simulink model "SLIPquadold"  (R2015a)
settings: Solver=ode45  StartTime=0.0  StopTime=50  MaxStep=1e-3  RelTol=1e-4  AbsTol=1e-6
values from neighbouring files (symbols this model uses):
  a0 = 68*pi/180    (= 1.18682389136)    [SLIPquad_params.m]
  dt0 = deg2rad(0)    [SLIPquad_params.m]
  dx0 = 4.5    [SLIPquad_params.m]
  dy0 = 0    [SLIPquad_params.m]
  g = 9.81    [SLIPquad_params.m]
  J = 4.58    [SLIPquad_params.m]
  Jleg = mfoot*l0^2    (= 1.16)    [SLIPquad_params.m]
  k = 10000    [SLIPquad_params.m]
  L = 0.5    [SLIPquad_params.m]
  l0 = 1    [SLIPquad_params.m]
  m = 80    [SLIPquad_params.m]
  t0 = 0*pi/180    (= 0)    [SLIPquad_params.m]
  x0 = 0    [SLIPquad_params.m]
  xrb0 = -l0*cos(a0) + L*cos(t0)    [SLIPquad_params.m]
  xrf0 = -l0*cos(a0) - L*cos(t0)    [SLIPquad_params.m]
  y0 = 1    [SLIPquad_params.m]
  yrb0 = l0*sin(a0) + L*sin(t0)    [SLIPquad_params.m]
  yrf0 = l0*sin(a0) - L*sin(t0)    [SLIPquad_params.m]
libraries: simulink_extras x2
settings Model: Creator=hgeyer  LastModifiedBy=Joe
settings DataIOCC: LimitDataPoints=off  SignalLoggingSaveFormat=ModelDataLogs
settings OptimizationCC: ExpressionDepthLimit=2147483647
settings DebuggingCC: UnderspecifiedInitializationDetection=Classic  MergeDetectMultiDrivingBlocksExec=none  SolverPrmCheckMsg=warning  FcnCallInpInsideContextMsg=EnableAllAsWarning  StateNameClashWarn=warning

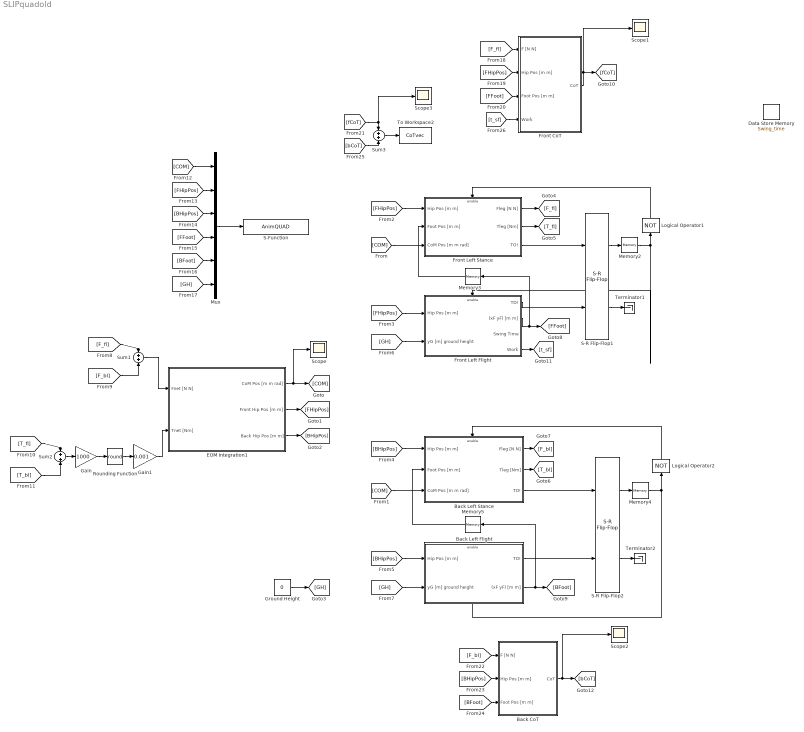
== system SLIPquadold ==
  Back CoT : Subsystem
  Back Left Flight : Subsystem
  Back Left Stance : Subsystem
  Data Store Memory : DataStoreMemory  DataStoreName=Swing_time  ReadBeforeWriteMsg=warning  WriteAfterWriteMsg=warning  WriteAfterReadMsg=warning
  EOM Integration1 : Subsystem
  Front CoT : Subsystem
  Front Left Flight : Subsystem
  Front Left Stance : Subsystem
  Gain : Gain  Gain=1000
  Gain1 : Gain  Gain=0.001
  Ground Height : Constant  Value=0
  Logical Operator1 : Logic  Operator=NOT  AllPortsSameDT=off  OutDataTypeStr=boolean
  Logical Operator2 : Logic  Operator=NOT  AllPortsSameDT=off  OutDataTypeStr=boolean
  Memory2 : Memory  X0=1
  Memory3 : Memory  X0=[(x0 - xrf0) (y0 - yrf0) ]
  Memory4 : Memory  X0=1
  Memory5 : Memory  X0=[(x0 - xrb0) (y0 - yrb0)]
  Mux : Mux  Inputs=6
  Rounding Function : Rounding  Operator=round
  S-Function : S-Function  FunctionName=AnimQUAD  Parameters=0.005
  S-R Flip-Flop1 : simulink_extras/Flip Flops/S-R Flip-Flop  initial_condition=1
  S-R Flip-Flop2 : simulink_extras/Flip Flops/S-R Flip-Flop  initial_condition=1
  Scope{,1..3} (4 alike) : Scope
      Scope2 settings: SaveName=ScopeData6
      Scope3 settings: SaveName=ScopeData7
  Sum1 : Sum  Inputs=+|+
  Sum2 : Sum  Inputs=+|+
  Sum3 : Sum  Inputs=+|+
  Terminator1 : Terminator
  Terminator2 : Terminator
  To Workspace2 : ToWorkspace  VariableName=CoTvec  SampleTime=-1
  wires:
  Front Left Stance/3(TO!) -> S-R Flip-Flop1/1
  S-R Flip-Flop1/1 -> Memory2/1
  Front Left Flight/1(TD!) -> S-R Flip-Flop1/2
  Memory2/1 -> Front Left Flight/Enable, Logical Operator1/1
  Logical Operator1/1 -> Front Left Stance/Enable
  S-R Flip-Flop1/2 -> Terminator1/1
  Front Left Flight/2((xF yF) [m m]) -> [FFoot], Memory3/1
  Memory3/1 -> Front Left Stance/2(Foot Pos [m m])
  Back Left Stance/3(TO!) -> S-R Flip-Flop2/1
  S-R Flip-Flop2/1 -> Memory4/1
  Back Left Flight/1(TO!) -> S-R Flip-Flop2/2
  Memory4/1 -> Back Left Flight/Enable, Logical Operator2/1
  Logical Operator2/1 -> Back Left Stance/Enable
  S-R Flip-Flop2/2 -> Terminator2/1
  [GH] -> Back Left Flight/2(yG [m] ground height)
  Back Left Flight/2((xF yF) [m m]) -> [BFoot], Memory5/1
  Memory5/1 -> Back Left Stance/2(Foot Pos [m m])
  Ground Height/1 -> [GH]
  [GH] -> Front Left Flight/2(yG [m] ground height)
  Front Left Stance/1(Fleg [N N]) -> [F_fl]
  Front Left Stance/2(Tleg [Nm]) -> [T_fl]
  Back Left Stance/1(Fleg [N N]) -> [F_bl]
  Back Left Stance/2(Tleg [Nm]) -> [T_bl]
  [F_fl] -> Sum1/1
  [F_bl] -> Sum1/2
  [T_fl] -> Sum2/1
  [T_bl] -> Sum2/2
  Sum1/1 -> EOM Integration1/1(Fnet [N N])
  EOM Integration1/1(CoM Pos [m m rad]) -> Scope/1, [COM]
  EOM Integration1/2(Front Hip Pos [m m]) -> [FHipPos]
  EOM Integration1/3(Back Hip Pos [m m]) -> [BHipPos]
  [FHipPos] -> Front Left Stance/1(Hip Pos [m m])
  [FHipPos] -> Front Left Flight/1(Hip Pos [m m])
  [BHipPos] -> Back Left Stance/1(Hip Pos [m m])
  [BHipPos] -> Back Left Flight/1(Hip Pos [m m])
  [COM] -> Front Left Stance/3(CoM Pos [m m rad])
  [COM] -> Back Left Stance/3(CoM Pos [m m rad])
  Sum2/1 -> Gain/1
  Gain1/1 -> EOM Integration1/2(Tnet [Nm])
  Gain/1 -> Rounding Function/1
  Rounding Function/1 -> Gain1/1
  Mux/1 -> S-Function/1
  [COM] -> Mux/1
  [FHipPos] -> Mux/2
  [BHipPos] -> Mux/3
  [FFoot] -> Mux/4
  [BFoot] -> Mux/5
  [GH] -> Mux/6
  [F_fl] -> Front CoT/1(F [N N])
  [FHipPos] -> Front CoT/2(Hip Pos [m m])
  [FFoot] -> Front CoT/3(Foot Pos [m m])
  Front CoT/1(CoT) -> [fCoT], Scope1/1
  [F_bl] -> Back CoT/1(F [N N])
  [BHipPos] -> Back CoT/2(Hip Pos [m m])
  [BFoot] -> Back CoT/3(Foot Pos [m m])
  Back CoT/1(CoT) -> [bCoT], Scope2/1
  [fCoT] -> Scope3/1, Sum3/1
  [bCoT] -> Sum3/2
  Sum3/1 -> To Workspace2/1
  [t_sf] -> Front CoT/4(Work)
  Front Left Flight/4(Work) -> [t_sf]

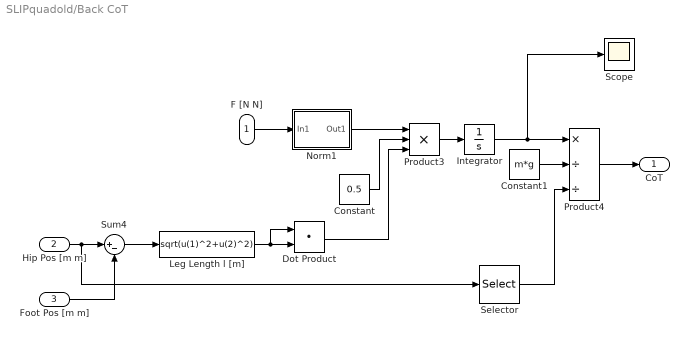
== system SLIPquadold/Back CoT ==
  F [N N] : Inport
  Hip Pos [m m] : Inport  Port=2
  Foot Pos [m m] : Inport  Port=3
  Constant : Constant  Value=0.5
  Constant1 : Constant  Value=m*g
  Dot Product : DotProduct  InputSameDT=on  OutDataTypeStr=Inherit: Inherit via internal rule
  Integrator : Integrator
  Leg Length l [m] : Fcn  Expr=sqrt(u(1)^2+u(2)^2)
  Norm1 : Subsystem
  Product3 : Product  Inputs=3
  Product4 : Product  Inputs=*//
  Scope : Scope
      settings: SaveName=ScopeData3
  Selector : Selector  InputPortWidth=2  Indices=[1]
  Sum4 : Sum  Inputs=|+-
  CoT : Outport
  wires:
  Constant/1 -> Product3/2
  Constant1/1 -> Product4/2
  Norm1/1(Out1) -> Product3/1
  Dot Product/1 -> Product3/3
  F [N N]/1 -> Norm1/1(In1)
  Leg Length l [m]/1 -> Dot Product/1, Dot Product/2
  Product4/1 -> CoT/1
  Product3/1 -> Integrator/1
  Selector/1 -> Product4/3
  Integrator/1 -> Scope/1, Product4/1
  Sum4/1 -> Leg Length l [m]/1
  Foot Pos [m m]/1 -> Sum4/2
  Hip Pos [m m]/1 -> Selector/1, Sum4/1

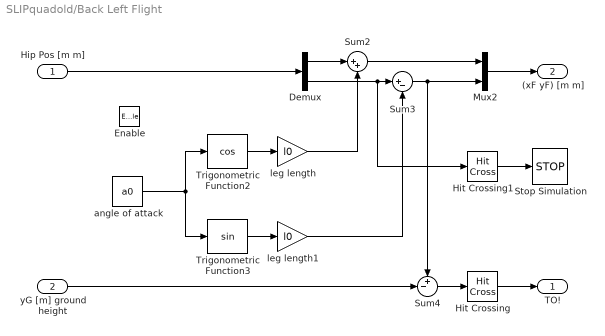
== system SLIPquadold/Back Left Flight ==
  Hip Pos [m m] : Inport
  yG [m] ground height : Inport  Port=2
  Enable : EnablePort  StatesWhenEnabling=reset
  Demux : Demux  Outputs=2
  Hit Crossing : HitCross  HitCrossingDirection=falling
  Hit Crossing1 : HitCross  HitCrossingDirection=falling
  Mux2 : Mux  Inputs=2
  Stop Simulation : Stop
  Sum2 : Sum  Inputs=|++
  Sum3 : Sum  Inputs=|+-
  Sum4 : Sum  Inputs=+-|
  Trigonometric Function2 : Trigonometry  Operator=cos
  Trigonometric Function3 : Trigonometry
  angle of attack : Constant  Value=a0
  leg length : Gain  Gain=l0
  leg length1 : Gain  Gain=l0
  TO! : Outport  OutputWhenDisabled=reset  InitialOutput=0
      settings: AttributesFormatString=%<OutputWhenDisabled>
  (xF yF) [m m] : Outport  Port=2  InitialOutput=[0 0]
      settings: AttributesFormatString=%<OutputWhenDisabled>
  wires:
  Hit Crossing/1 -> TO!/1
  Demux/2 -> Hit Crossing1/1, Sum3/1
  Demux/1 -> Sum2/1
  angle of attack/1 -> Trigonometric Function3/1, Trigonometric Function2/1
  Trigonometric Function2/1 -> leg length/1
  Trigonometric Function3/1 -> leg length1/1
  Hip Pos [m m]/1 -> Demux/1
  leg length/1 -> Sum2/2
  leg length1/1 -> Sum3/2
  Sum3/1 -> Mux2/2, Sum4/1
  Sum2/1 -> Mux2/1
  Mux2/1 -> (xF yF) [m m]/1
  yG [m] ground height/1 -> Sum4/2
  Sum4/1 -> Hit Crossing/1
  Hit Crossing1/1 -> Stop Simulation/1

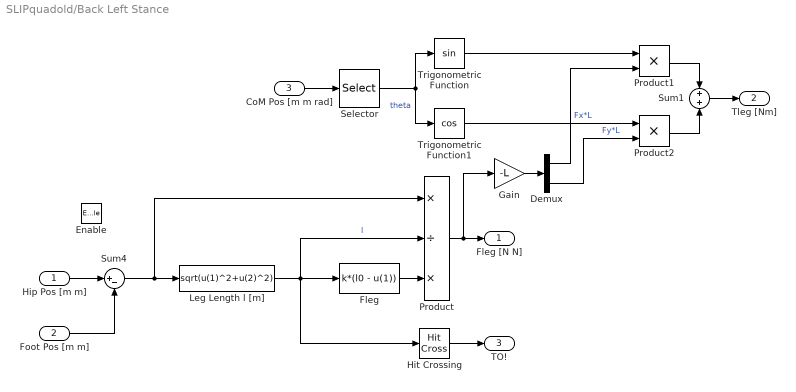
== system SLIPquadold/Back Left Stance ==
  Hip Pos [m m] : Inport
  Foot Pos [m m] : Inport  Port=2
  CoM Pos [m m rad] : Inport  Port=3
  Enable : EnablePort  StatesWhenEnabling=reset
  Demux : Demux  Outputs=2
  Fleg : Fcn  Expr=k*(l0 - u(1))
  Gain : Gain  Gain=-L
  Hit Crossing : HitCross  HitCrossingOffset=l0  HitCrossingDirection=rising
  Leg Length l [m] : Fcn  Expr=sqrt(u(1)^2+u(2)^2)
  Product : Product  Inputs=*/*
  Product1 : Product
  Product2 : Product
  Selector : Selector  InputPortWidth=3  Indices=[3]
  Sum1 : Sum  Inputs=+|+
  Sum4 : Sum  Inputs=|+-
  Trigonometric Function : Trigonometry
  Trigonometric Function1 : Trigonometry  Operator=cos
  Fleg [N N] : Outport  OutputWhenDisabled=reset  InitialOutput=[0 0]
      settings: AttributesFormatString=%<OutputWhenDisabled>
  Tleg [Nm] : Outport  Port=2  OutputWhenDisabled=reset  InitialOutput=[0]
      settings: AttributesFormatString=%<OutputWhenDisabled>
  TO! : Outport  Port=3  OutputWhenDisabled=reset  InitialOutput=[0]
      settings: AttributesFormatString=%<OutputWhenDisabled>
  wires:
  Sum1/1 -> Tleg [Nm]/1
  Product1/1 -> Sum1/1
  Product2/1 -> Sum1/2
  Gain/1 -> Demux/1
  Demux/2 -> Product2/2  "Fy*L"
  Demux/1 -> Product1/2  "Fx*L"
  Trigonometric Function/1 -> Product1/1
  Trigonometric Function1/1 -> Product2/1
  Selector/1 -> Trigonometric Function/1, Trigonometric Function1/1  "theta"
  CoM Pos [m m rad]/1 -> Selector/1
  Foot Pos [m m]/1 -> Sum4/2
  Hip Pos [m m]/1 -> Sum4/1
  Hit Crossing/1 -> TO!/1
  Product/1 -> Fleg [N N]/1, Gain/1
  Fleg/1 -> Product/3
  Leg Length l [m]/1 -> Hit Crossing/1, Product/2, Fleg/1  "l"
  Sum4/1 -> Leg Length l [m]/1, Product/1

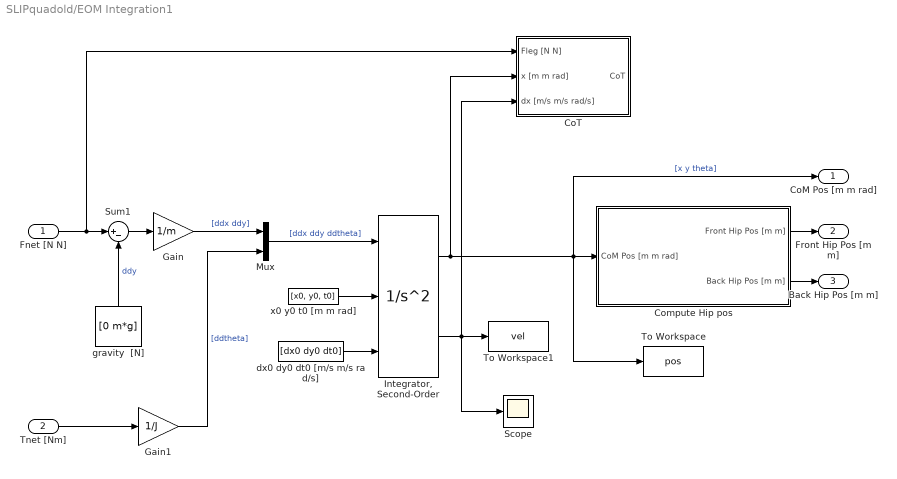
== system SLIPquadold/EOM Integration1 ==
  Fnet [N N] : Inport
  Tnet [Nm] : Inport  Port=2
  CoT : Subsystem
  Compute Hip pos : Subsystem
  Gain : Gain  Gain=1/m
  Gain1 : Gain  Gain=1/J
  "Integrator, Second-Order" : SecondOrderIntegrator  ICSourceX=external  ICSourceDXDT=external
  Mux : Mux  Inputs=2
  Scope : Scope
      settings: TimeRange=3.298211913921595  YMin=-10  YMax=10  SaveName=ScopeData2
  Sum1 : Sum  Inputs=|+-
  To Workspace : ToWorkspace  VariableName=pos  SampleTime=-1
  To Workspace1 : ToWorkspace  VariableName=vel  SampleTime=-1
  dx0 dy0 dt0 [m/s m/s ra d/s] : Constant  Value=[dx0 dy0 dt0]
  gravity  [N] : Constant  Value=[0 m*g]
  x0 y0 t0 [m m rad] : Constant  Value=[x0, y0, t0]
  CoM Pos [m m rad] : Outport
  Front Hip Pos [m m] : Outport  Port=2
  Back Hip Pos [m m] : Outport  Port=3
  wires:
  "Integrator, Second-Order"/2 -> CoT/3(dx [m/s m/s rad/s]), Scope/1, To Workspace1/1
  Compute Hip pos/1(Front Hip Pos [m m]) -> Front Hip Pos [m m]/1
  "Integrator, Second-Order"/1 -> CoT/2(x [m m rad]), CoM Pos [m m rad]/1, Compute Hip pos/1(CoM Pos [m m rad]), To Workspace/1  "[x y theta]"
  Tnet [Nm]/1 -> Gain1/1
  Gain1/1 -> Mux/2  "[ddtheta]"
  Mux/1 -> "Integrator, Second-Order"/1  "[ddx ddy ddtheta]"
  dx0 dy0 dt0 [m/s m/s ra d/s]/1 -> "Integrator, Second-Order"/3
  Fnet [N N]/1 -> CoT/1(Fleg [N N]), Sum1/1
  Gain/1 -> Mux/1  "[ddx ddy]"
  x0 y0 t0 [m m rad]/1 -> "Integrator, Second-Order"/2
  gravity  [N]/1 -> Sum1/2  "ddy"
  Sum1/1 -> Gain/1
  Compute Hip pos/2(Back Hip Pos [m m]) -> Back Hip Pos [m m]/1

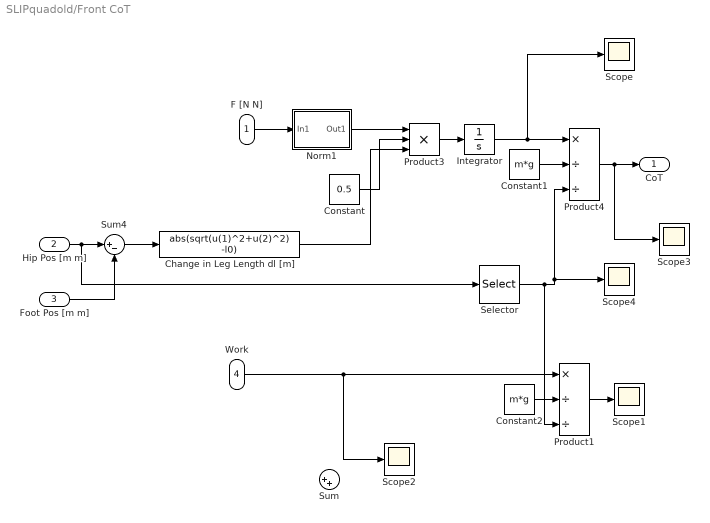
== system SLIPquadold/Front CoT ==
  F [N N] : Inport
  Hip Pos [m m] : Inport  Port=2
  Foot Pos [m m] : Inport  Port=3
  Work : Inport  Port=4
  Change in Leg Length dl [m] : Fcn  Expr=abs(sqrt(u(1)^2+u(2)^2) -l0)
  Constant : Constant  Value=0.5
  Constant1 : Constant  Value=m*g
  Constant2 : Constant  Value=m*g
  Integrator : Integrator
  Norm1 : Subsystem
  Product1 : Product  Inputs=*//
  Product3 : Product  Inputs=3
  Product4 : Product  Inputs=*//
  Scope{,1..4} (5 alike) : Scope
      Scope settings: YMin=2000  YMax=6000  SaveName=ScopeData3
      Scope1 settings: SaveName=ScopeData8
      Scope2 settings: SaveName=ScopeData9
      Scope3 settings: YMin=0.0443  YMax=0.04445  SaveName=ScopeData10
      Scope4 settings: YMin=2000  YMax=6000  SaveName=ScopeData12
  Selector : Selector  InputPortWidth=2  Indices=[1]
  Sum : Sum  Inputs=|++
  Sum4 : Sum  Inputs=|+-
  CoT : Outport
  wires:
  Constant/1 -> Product3/2
  Constant1/1 -> Product4/2
  Norm1/1(Out1) -> Product3/1
  F [N N]/1 -> Norm1/1(In1)
  Product4/1 -> Scope3/1, CoT/1
  Product3/1 -> Integrator/1
  Selector/1 -> Product1/3, Product4/3, Scope4/1
  Integrator/1 -> Scope/1, Product4/1
  Sum4/1 -> Change in Leg Length dl [m]/1
  Foot Pos [m m]/1 -> Sum4/2
  Hip Pos [m m]/1 -> Selector/1, Sum4/1
  Constant2/1 -> Product1/2
  Product1/1 -> Scope1/1
  Work/1 -> Product1/1, Scope2/1
  Change in Leg Length dl [m]/1 -> Product3/3

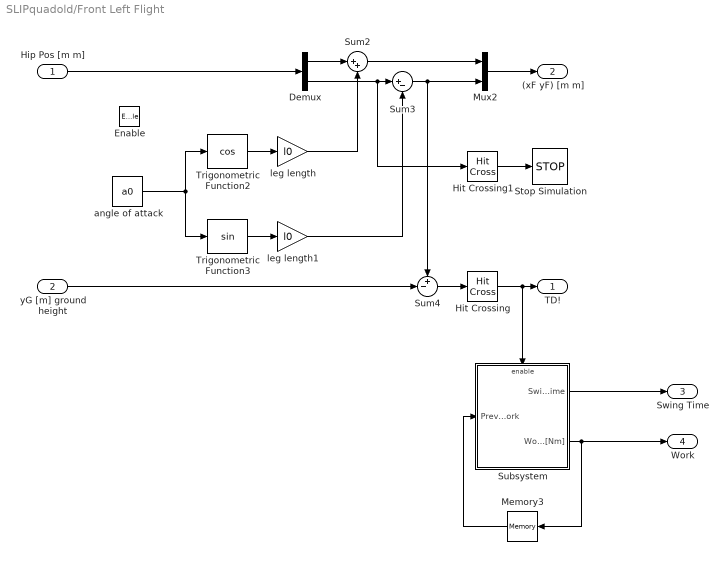
== system SLIPquadold/Front Left Flight ==
  Hip Pos [m m] : Inport
  yG [m] ground height : Inport  Port=2
  Enable : EnablePort  StatesWhenEnabling=reset
  Demux : Demux  Outputs=2
  Hit Crossing : HitCross  HitCrossingDirection=falling
  Hit Crossing1 : HitCross  HitCrossingDirection=falling
  Memory3 : Memory  X0=[(x0 - xrf0) (y0 - yrf0) ]
  Mux2 : Mux  Inputs=2
  Stop Simulation : Stop
  Subsystem : Subsystem
  Sum2 : Sum  Inputs=|++
  Sum3 : Sum  Inputs=|+-
  Sum4 : Sum  Inputs=+-|
  Trigonometric Function2 : Trigonometry  Operator=cos
  Trigonometric Function3 : Trigonometry
  angle of attack : Constant  Value=a0
  leg length : Gain  Gain=l0
  leg length1 : Gain  Gain=l0
  TD! : Outport  OutputWhenDisabled=reset  InitialOutput=0
      settings: AttributesFormatString=%<OutputWhenDisabled>
  (xF yF) [m m] : Outport  Port=2  InitialOutput=[0 0]
      settings: AttributesFormatString=%<OutputWhenDisabled>
  Swing Time : Outport  Port=3  OutputWhenDisabled=reset  InitialOutput=0
      settings: AttributesFormatString=%<OutputWhenDisabled>
  Work : Outport  Port=4  InitialOutput=0
      settings: AttributesFormatString=%<OutputWhenDisabled>
  wires:
  Hit Crossing1/1 -> Stop Simulation/1
  Sum4/1 -> Hit Crossing/1
  yG [m] ground height/1 -> Sum4/2
  Mux2/1 -> (xF yF) [m m]/1
  Sum2/1 -> Mux2/1
  Sum3/1 -> Sum4/1, Mux2/2
  leg length1/1 -> Sum3/2
  leg length/1 -> Sum2/2
  Hip Pos [m m]/1 -> Demux/1
  Trigonometric Function3/1 -> leg length1/1
  Trigonometric Function2/1 -> leg length/1
  angle of attack/1 -> Trigonometric Function2/1, Trigonometric Function3/1
  Demux/1 -> Sum2/1
  Demux/2 -> Sum3/1, Hit Crossing1/1
  Hit Crossing/1 -> TD!/1, Subsystem/Enable
  Subsystem/1(Swing Time) -> Swing Time/1
  Subsystem/2(Work [Nm]) -> Work/1, Memory3/1
  Memory3/1 -> Subsystem/1(Previous Work)

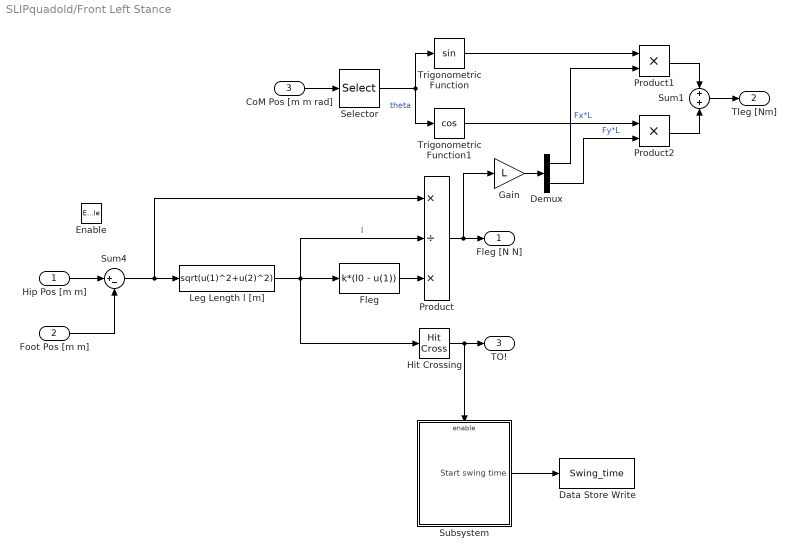
== system SLIPquadold/Front Left Stance ==
  Hip Pos [m m] : Inport
  Foot Pos [m m] : Inport  Port=2
  CoM Pos [m m rad] : Inport  Port=3
  Enable : EnablePort  StatesWhenEnabling=reset
  Data Store Write : DataStoreWrite  DataStoreName=Swing_time
  Demux : Demux  Outputs=2
  Fleg : Fcn  Expr=k*(l0 - u(1))
  Gain : Gain  Gain=L
  Hit Crossing : HitCross  HitCrossingOffset=l0  HitCrossingDirection=rising
  Leg Length l [m] : Fcn  Expr=sqrt(u(1)^2+u(2)^2)
  Product : Product  Inputs=*/*
  Product1 : Product
  Product2 : Product
  Selector : Selector  InputPortWidth=3  Indices=[3]
  Subsystem : Subsystem
  Sum1 : Sum  Inputs=+|+
  Sum4 : Sum  Inputs=|+-
  Trigonometric Function : Trigonometry
  Trigonometric Function1 : Trigonometry  Operator=cos
  Fleg [N N] : Outport  OutputWhenDisabled=reset  InitialOutput=[0 0]
      settings: AttributesFormatString=%<OutputWhenDisabled>
  Tleg [Nm] : Outport  Port=2  OutputWhenDisabled=reset  InitialOutput=[0]
      settings: AttributesFormatString=%<OutputWhenDisabled>
  TO! : Outport  Port=3  OutputWhenDisabled=reset  InitialOutput=[0]
      settings: AttributesFormatString=%<OutputWhenDisabled>
  wires:
  Sum4/1 -> Product/1, Leg Length l [m]/1
  Leg Length l [m]/1 -> Fleg/1, Product/2, Hit Crossing/1  "l"
  Fleg/1 -> Product/3
  Product/1 -> Fleg [N N]/1, Gain/1
  Hit Crossing/1 -> Subsystem/Enable, TO!/1
  Hip Pos [m m]/1 -> Sum4/1
  Foot Pos [m m]/1 -> Sum4/2
  CoM Pos [m m rad]/1 -> Selector/1
  Selector/1 -> Trigonometric Function1/1, Trigonometric Function/1  "theta"
  Trigonometric Function1/1 -> Product2/1
  Trigonometric Function/1 -> Product1/1
  Demux/1 -> Product1/2  "Fx*L"
  Demux/2 -> Product2/2  "Fy*L"
  Gain/1 -> Demux/1
  Product2/1 -> Sum1/2
  Product1/1 -> Sum1/1
  Sum1/1 -> Tleg [Nm]/1
  Subsystem/1(Start swing time) -> Data Store Write/1

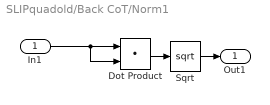
== system SLIPquadold/Back CoT/Norm1 ==
  In1 : Inport
  Dot Product : DotProduct  InputSameDT=on  OutDataTypeStr=Inherit: Inherit via internal rule
  Sqrt : Sqrt  SaturateOnIntegerOverflow=on
  Out1 : Outport
  wires:
  Sqrt/1 -> Out1/1
  In1/1 -> Dot Product/2, Dot Product/1
  Dot Product/1 -> Sqrt/1

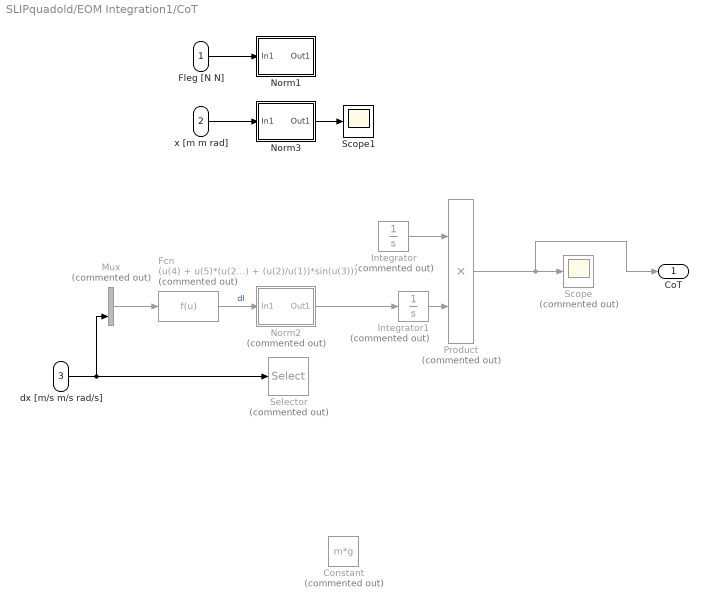
== system SLIPquadold/EOM Integration1/CoT ==
  Fleg [N N] : Inport
  x [m m rad] : Inport  Port=2
  dx [m/s m/s rad/s] : Inport  Port=3
  Constant : Constant  Commented=on  Value=m*g
  Fcn : Fcn  Commented=on  Expr=(u(4) + u(5)*(u(2)/u(1)))/(cos(u(3)) + (u(2)/u(1))*sin(u(3)))
  Integrator : Integrator  Commented=on
  Integrator1 : Integrator  Commented=on
  Mux : Mux  Commented=on  Inputs=2
  Norm1 : Subsystem
  Norm2 : Subsystem  Commented=on
  Norm3 : Subsystem
  Product : Product  Commented=on  Inputs=**
  Scope : Scope  Commented=on
      settings: SaveName=ScopeData4
  Scope1 : Scope
      settings: SaveName=ScopeData5
  Selector : Selector  Commented=on  InputPortWidth=3  Indices=[1]
  CoT : Outport
  wires:
  Norm2/1(Out1) -> Integrator1/1
  Fleg [N N]/1 -> Norm1/1(In1)
  dx [m/s m/s rad/s]/1 -> Selector/1, Mux/2
  ? -> Mux/1
  Mux/1 -> Fcn/1
  Fcn/1 -> Norm2/1(In1)  "dl"
  Product/1 -> CoT/1, Scope/1
  Integrator/1 -> Product/1
  Integrator1/1 -> Product/2
  x [m m rad]/1 -> Norm3/1(In1)
  Norm3/1(Out1) -> Scope1/1

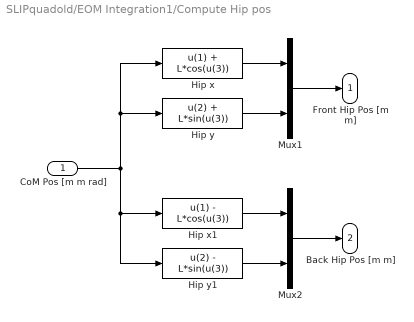
== system SLIPquadold/EOM Integration1/Compute Hip pos ==
  CoM Pos [m m rad] : Inport
  Hip x : Fcn  Expr=u(1) + L*cos(u(3))
  Hip x1 : Fcn  Expr=u(1) - L*cos(u(3))
  Hip y : Fcn  Expr=u(2) + L*sin(u(3))
  Hip y1 : Fcn  Expr=u(2) - L*sin(u(3))
  Mux1 : Mux  Inputs=2
  Mux2 : Mux  Inputs=2
  Front Hip Pos [m m] : Outport
  Back Hip Pos [m m] : Outport  Port=2
  wires:
  Hip y/1 -> Mux1/2
  Mux1/1 -> Front Hip Pos [m m]/1
  Hip x/1 -> Mux1/1
  Hip y1/1 -> Mux2/2
  Mux2/1 -> Back Hip Pos [m m]/1
  Hip x1/1 -> Mux2/1
  CoM Pos [m m rad]/1 -> Hip x/1, Hip y/1, Hip y1/1, Hip x1/1

== system SLIPquadold/Front CoT/Norm1 ==
  In1 : Inport
  Dot Product : DotProduct  InputSameDT=on  OutDataTypeStr=Inherit: Inherit via internal rule
  Sqrt : Sqrt  SaturateOnIntegerOverflow=on
  Out1 : Outport
  wires:
  Sqrt/1 -> Out1/1
  In1/1 -> Dot Product/2, Dot Product/1
  Dot Product/1 -> Sqrt/1

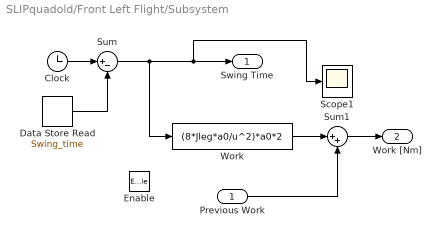
== system SLIPquadold/Front Left Flight/Subsystem ==
  Previous Work : Inport
  Enable : EnablePort  StatesWhenEnabling=reset
  Clock : Clock
  Data Store Read : DataStoreRead  DataStoreName=Swing_time
  Scope1 : Scope
      settings: SaveName=ScopeData11
  Sum : Sum  Inputs=|+-
  Sum1 : Sum  Inputs=|++
  Work : Fcn  Expr=(8*Jleg*a0/u^2)*a0*2
  Swing Time : Outport  OutputWhenDisabled=reset  InitialOutput=0
      settings: AttributesFormatString=%<OutputWhenDisabled>
  Work [Nm] : Outport  Port=2  InitialOutput=0
      settings: AttributesFormatString=%<OutputWhenDisabled>
  wires:
  Sum/1 -> Work/1, Scope1/1, Swing Time/1
  Clock/1 -> Sum/1
  Data Store Read/1 -> Sum/2
  Work/1 -> Sum1/1
  Sum1/1 -> Work [Nm]/1
  Previous Work/1 -> Sum1/2

== system SLIPquadold/Front Left Stance/Subsystem ==
  Enable : EnablePort  StatesWhenEnabling=reset
  Clock : Clock
  Start swing time : Outport  InitialOutput=0
      settings: AttributesFormatString=%<OutputWhenDisabled>
  wires:
  Clock/1 -> Start swing time/1

== system SLIPquadold/EOM Integration1/CoT/Norm1 ==
  In1 : Inport
  Dot Product : DotProduct  InputSameDT=on  OutDataTypeStr=Inherit: Inherit via internal rule
  Sqrt : Sqrt  SaturateOnIntegerOverflow=on
  Out1 : Outport
  wires:
  Sqrt/1 -> Out1/1
  In1/1 -> Dot Product/2, Dot Product/1
  Dot Product/1 -> Sqrt/1

== system SLIPquadold/EOM Integration1/CoT/Norm2 ==
  In1 : Inport
  Dot Product : DotProduct  InputSameDT=on  OutDataTypeStr=Inherit: Inherit via internal rule
  Sqrt : Sqrt  SaturateOnIntegerOverflow=on
  Out1 : Outport
  wires:
  Dot Product/1 -> Sqrt/1
  In1/1 -> Dot Product/1, Dot Product/2
  Sqrt/1 -> Out1/1

== system SLIPquadold/EOM Integration1/CoT/Norm3 ==
  In1 : Inport
  Dot Product : DotProduct  InputSameDT=on  OutDataTypeStr=Inherit: Inherit via internal rule
  Sqrt : Sqrt  SaturateOnIntegerOverflow=on
  Out1 : Outport
  wires:
  Dot Product/1 -> Sqrt/1
  In1/1 -> Dot Product/1, Dot Product/2
  Sqrt/1 -> Out1/1
